simulink model "Wiper_New_Harness5"  (R2022b)
settings: Solver=FixedStepAuto  StartTime=0.0  StopTime=10.0  FixedStep=0.01  RelTol=1e-3
settings Model: Creator=suha274823  LastModifiedBy=suha274823
settings ConfigComp: CovEnable=on  RecordCoverage=on  CovSaveSingleToWorkspaceVar=on  CovModelRefEnable=on

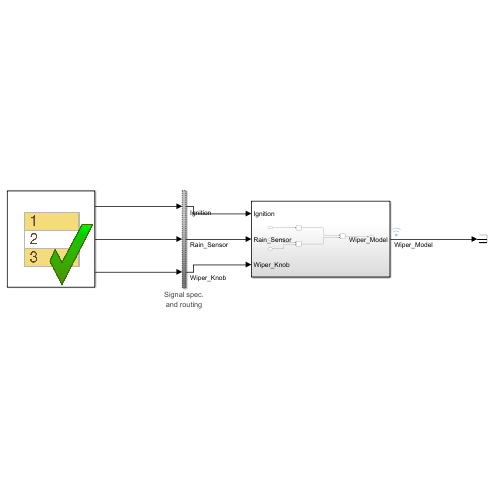
[thumbnail: Simulink's stored preview of the top-level diagram]
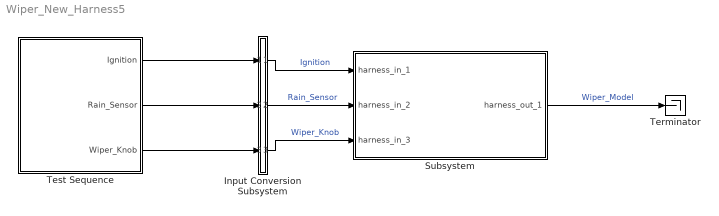
== system Wiper_New_Harness5 ==
  Input Conversion Subsystem : Subsystem  Tag=__SLT_ICS__  Description=|
      | Signal spec.
      | and routing
      settings: AttributesFormatString=%<Description>
  Subsystem : Subsystem  Tag=__SL_testing_harness_stub_
  Terminator : Terminator
  Test Sequence : Test Sequence  TreatAsAtomicUnit=on
  wires:
  Test Sequence/1(Ignition) -> Input Conversion Subsystem/1(Inport_1)
  Test Sequence/2(Rain_Sensor) -> Input Conversion Subsystem/2(Inport_2)
  Test Sequence/3(Wiper_Knob) -> Input Conversion Subsystem/3(Inport_3)
  Input Conversion Subsystem/1(Outport_1) -> Subsystem/1(harness_in_1)  "Ignition"
  Input Conversion Subsystem/2(Outport_2) -> Subsystem/2(harness_in_2)  "Rain_Sensor"
  Input Conversion Subsystem/3(Outport_3) -> Subsystem/3(harness_in_3)  "Wiper_Knob"
  Subsystem/1(harness_out_1) -> Terminator/1  "Wiper_Model"

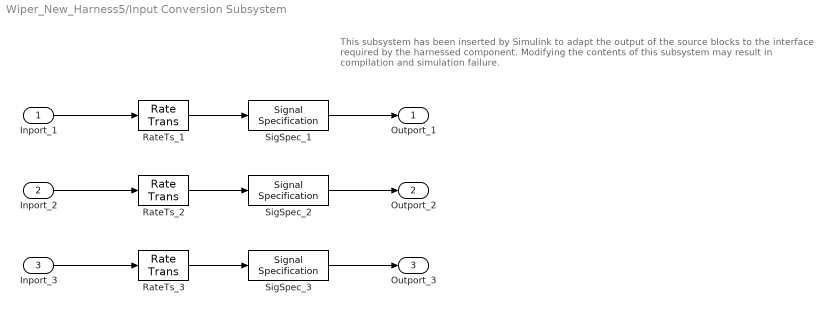
== system Wiper_New_Harness5/Input Conversion Subsystem ==
  note: This subsystem has been inserted by Simulink to adapt the output of the source blocks to the interface required by the harnessed component.
      |  Modifying the contents of this subsystem may result in compilation and simulation failure.
  Inport_1 : Inport
  Inport_2 : Inport  Port=2
  Inport_3 : Inport  Port=3
  RateTs_1 : RateTransition  OutPortSampleTime=0.01
  RateTs_2 : RateTransition  OutPortSampleTime=0.01
  RateTs_3 : RateTransition  OutPortSampleTime=0.01
  SigSpec_1 : SignalSpecification  OutDataTypeStr=double  Dimensions=[1]  SampleTime=0.01
  SigSpec_2 : SignalSpecification  OutDataTypeStr=boolean  Dimensions=[1]  SampleTime=0.01
  SigSpec_3 : SignalSpecification  OutDataTypeStr=boolean  Dimensions=[1]  SampleTime=0.01
  Outport_1 : Outport
  Outport_2 : Outport  Port=2
  Outport_3 : Outport  Port=3
  wires:
  SigSpec_1/1 -> Outport_1/1
  RateTs_1/1 -> SigSpec_1/1
  Inport_1/1 -> RateTs_1/1
  SigSpec_2/1 -> Outport_2/1
  RateTs_2/1 -> SigSpec_2/1
  Inport_2/1 -> RateTs_2/1
  SigSpec_3/1 -> Outport_3/1
  RateTs_3/1 -> SigSpec_3/1
  Inport_3/1 -> RateTs_3/1

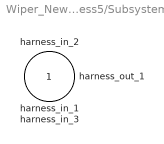
== system Wiper_New_Harness5/Subsystem ==
  harness_in_1 : Inport
  harness_in_2 : Inport  Port=2
  harness_in_3 : Inport  Port=3
  harness_out_1 : Outport

== stateflow chart Wiper_New_Harness5/Test Sequence ==
  settings: updateMethod=DISCRETE  sampleTime=0.01
  state TC_05
    %% Initialize data outputs.
    Ignition = 0;
    Rain_Sensor = true;
    Wiper_Knob = true;
  (default) -> TC_05
  data: Ignition output double size=[1]; Rain_Sensor output boolean size=[1]; Wiper_Knob output boolean size=[1]
